simulink model "distributed_system"  (R2018a)
settings: Solver=VariableStepDiscrete  StartTime=0.0  StopTime=Inf  FixedStep=0.01  RelTol=1e-3  EnableMultiTasking=on
model workspace (MAT data in the model file):
  SL_ROS_VariableLengthArrays_MaxSizes.CommonInfo.ArrayTruncateAction = 'EmitWarning'
  SL_ROS_VariableLengthArrays_MaxSizes.MsgTypeMap = containers.Map
  SL_ROS_VariableLengthArrays_MaxSizes.MsgTypeMap.serialization.keys = {'sensor_msgs/Image', 'sensor_msgs/LaserScan'}
  SL_ROS_VariableLengthArrays_MaxSizes.MsgTypeMap.serialization.values{1}(1).PropertyName = 'Data'
  SL_ROS_VariableLengthArrays_MaxSizes.MsgTypeMap.serialization.values{1}(1).DataType = 'uint8'
  SL_ROS_VariableLengthArrays_MaxSizes.MsgTypeMap.serialization.values{1}(1).MaxLength = 691200
  SL_ROS_VariableLengthArrays_MaxSizes.MsgTypeMap.serialization.values{1}(2).PropertyName = 'Encoding'
  SL_ROS_VariableLengthArrays_MaxSizes.MsgTypeMap.serialization.values{1}(2).DataType = 'uint8'
  SL_ROS_VariableLengthArrays_MaxSizes.MsgTypeMap.serialization.values{1}(2).MaxLength = 128
  SL_ROS_VariableLengthArrays_MaxSizes.MsgTypeMap.serialization.values{2}(1).PropertyName = 'Intensities'
  SL_ROS_VariableLengthArrays_MaxSizes.MsgTypeMap.serialization.values{2}(1).DataType = 'single'
  SL_ROS_VariableLengthArrays_MaxSizes.MsgTypeMap.serialization.values{2}(1).MaxLength = 1081
  SL_ROS_VariableLengthArrays_MaxSizes.MsgTypeMap.serialization.values{2}(2).PropertyName = 'Ranges'
  SL_ROS_VariableLengthArrays_MaxSizes.MsgTypeMap.serialization.values{2}(2).DataType = 'single'
  SL_ROS_VariableLengthArrays_MaxSizes.MsgTypeMap.serialization.values{2}(2).MaxLength = 1081
  SL_ROS_VariableLengthArrays_MaxSizes.MsgTypeMap.serialization.uniformity = 0
  SL_ROS_VariableLengthArrays_MaxSizes.MsgTypeMap.serialization.keyType = 'char'
  SL_ROS_VariableLengthArrays_MaxSizes.MsgTypeMap.serialization.valueType = 'any'
undefined symbols (not defined in the file or in its folder): DiscIntNeverNeededParam, hz, Vector_
libraries: simulink x5, robotlib x4, sharedTrackingLibrary x4, aerolibanimutils x1
settings Model: Creator=The MathWorks, Inc.  LastModifiedBy=kevin
settings DataIOCC: LimitDataPoints=on  SaveFormat=Array
settings OptimizationCC: LifeSpan=Inf  MaxStackSize=64
settings DebuggingCC: SolverPrmCheckMsg=warning  SFUnexpectedBacktrackingDiag=warning  SFNoUnconditionalDefaultTransitionDiag=warning  SFExecutionAtInitializationDiag=none
settings HardwareCC: ProdBitPerLong=64  ProdHWDeviceType=Intel->x86-64 (Linux 64)  UseEmbeddedCoderFeatures=off
settings ModelReferenceCC: PropagateSignalLabelsOutOfModel=off
settings RTWCC: SystemTargetFile=ert.tlc  HardwareBoard=Robot Operating System (ROS)  TLCOptions=-aInlineSetEventsForThisBaseRateFcn=TLC_FALSE -aSuppressMultiTaskScheduler=TLC_FALSE -aRateBasedStepFcn=0  TemplateMakefile=ert_default_tmf  Toolchain=Catkin  TargetLang=C++
settings CodeAppCC: StateflowObjectComments=on
settings ERTTargetCC: MultiwordLength=2048  ERTCustomFileBanners=off  SupportContinuousTime=on  SupportNonInlinedSFcns=on  RemoveResetFunc=off  SupportVariableSizeSignals=on  ModelStepFunctionPrototypeControlCompliant=off  ConvertIfToSwitch=off  SuppressUnreachableDefaultCases=off
settings ConfigComp: CovMetricSettings=dw  CovHtmlReporting=on  CovSaveCumulativeToWorkspaceVar=on  CovSaveSingleToWorkspaceVar=on  CovExternalEMLEnable=off  CovSFcnEnable=off

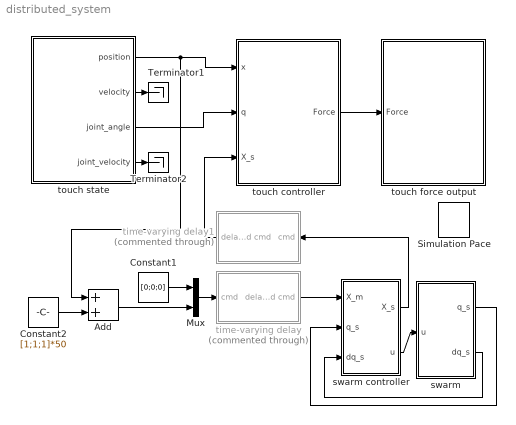
== system distributed_system ==
  Add : Sum
  Constant1 : Constant  Value=[0;0;0]
  Constant2 : Constant  Value=[1;1;1]*50
  Mux : Mux  Inputs=2
  Simulation Pace : aerolibanimutils/Simulation Pace  SimulationPace=1  SleepMode=MATLAB Thread  OutputPaceError=off  SampleTime=-1
  Terminator1 : Terminator
  Terminator2 : Terminator
  swarm : Subsystem
  swarm controller : Subsystem
  time-varying delay : Subsystem  Commented=through
  time-varying delay1 : Subsystem  Commented=through
  touch controller : Subsystem
  touch force output : Subsystem
  touch state : Subsystem
  wires:
  swarm/1(q_s) -> swarm controller/2(q_s)
  swarm/2(dq_s) -> swarm controller/3(dq_s)
  swarm controller/2(u) -> swarm/1(u)
  touch controller/1(Force) -> touch force output/1(Force)
  touch state/3(joint_angle) -> touch controller/2(q)
  swarm controller/1(X_s) -> time-varying delay1/1(cmd)
  Mux/1 -> time-varying delay/1(cmd)
  time-varying delay/1(delayed cmd) -> swarm controller/1(X_m)
  time-varying delay1/1(delayed cmd) -> touch controller/3(X_s)
  touch state/2(velocity) -> Terminator1/1
  touch state/4(joint_velocity) -> Terminator2/1
  Constant1/1 -> Mux/1
  Constant2/1 -> Add/2
  touch state/1(position) -> Add/1, touch controller/1(x)
  Add/1 -> Mux/2

== system distributed_system/swarm ==
  u : Inport
  Discrete-Time Integrator : DiscreteIntegrator  InitialCondition=zeros(18,1)  SampleTime=-1  ICPrevOutput=DiscIntNeverNeededParam  ICPrevScaledInput=DiscIntNeverNeededParam
  Discrete-Time Integrator1 : DiscreteIntegrator  InitialCondition=[1 0 0 0.7 0.7 0 -0.7 0.7 0 -1 0 0 -0.7 -0.7 0 0.7 -0.7 0].'  SampleTime=-1  ICPrevOutput=DiscIntNeverNeededParam  ICPrevScaledInput=DiscIntNeverNeededParam
  Subsystem1 : Subsystem
  q_s : Outport
  dq_s : Outport  Port=2
  wires:
  u/1 -> Discrete-Time Integrator/1
  Discrete-Time Integrator/1 -> Discrete-Time Integrator1/1, dq_s/1
  Discrete-Time Integrator1/1 -> q_s/1, Subsystem1/1(In1)

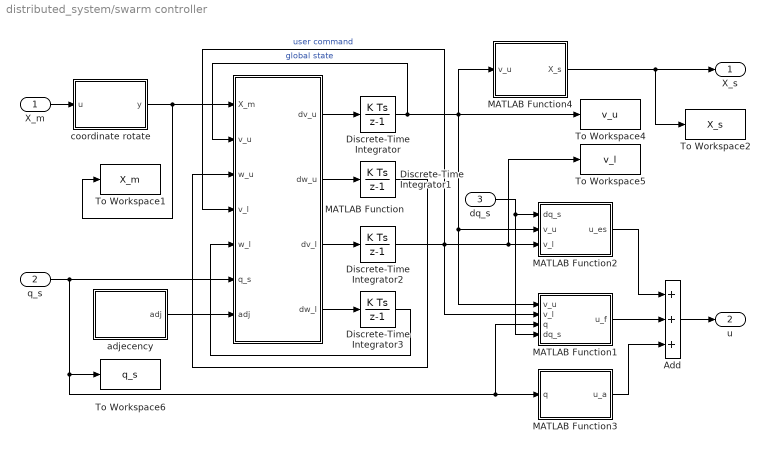
== system distributed_system/swarm controller ==
  X_m : Inport
  q_s : Inport  Port=2
  dq_s : Inport  Port=3
  Add : Sum  Inputs=+++
  Discrete-Time Integrator{,1..3} (4 alike) : DiscreteIntegrator  SampleTime=-1  ICPrevOutput=DiscIntNeverNeededParam  ICPrevScaledInput=DiscIntNeverNeededParam
  MATLAB Function : MATLAB Function  TreatAsAtomicUnit=on
  MATLAB Function1 : MATLAB Function  TreatAsAtomicUnit=on
  MATLAB Function2 : MATLAB Function  TreatAsAtomicUnit=on
  MATLAB Function3 : MATLAB Function  TreatAsAtomicUnit=on
  MATLAB Function4 : MATLAB Function  TreatAsAtomicUnit=on
  To Workspace1 : ToWorkspace  VariableName=X_m  SampleTime=-1
  To Workspace2 : ToWorkspace  VariableName=X_s  SampleTime=-1
  To Workspace4 : ToWorkspace  VariableName=v_u  SampleTime=-1
  To Workspace5 : ToWorkspace  VariableName=v_l  SampleTime=-1
  To Workspace6 : ToWorkspace  VariableName=q_s  SampleTime=-1
  adjecency : MATLAB Function  TreatAsAtomicUnit=on
  coordinate rotate : MATLAB Function  TreatAsAtomicUnit=on
  X_s : Outport
  u : Outport  Port=2
  wires:
  Discrete-Time Integrator1/1 -> MATLAB Function/3(w_u)
  q_s/1 -> MATLAB Function1/3(q), MATLAB Function3/1(q), To Workspace6/1, MATLAB Function/6(q_s)
  Discrete-Time Integrator3/1 -> MATLAB Function/5(w_l)
  Discrete-Time Integrator2/1 -> To Workspace5/1, MATLAB Function2/3(v_l), MATLAB Function1/2(v_l), MATLAB Function/4(v_l)  "user command"
  MATLAB Function/3(dv_l) -> Discrete-Time Integrator2/1
  MATLAB Function/4(dw_l) -> Discrete-Time Integrator3/1
  Add/1 -> u/1
  MATLAB Function/2(dw_u) -> Discrete-Time Integrator1/1
  Discrete-Time Integrator/1 -> To Workspace4/1, MATLAB Function4/1(v_u), MATLAB Function1/1(v_u), MATLAB Function2/2(v_u), MATLAB Function/2(v_u)  "global state"
  MATLAB Function/1(dv_u) -> Discrete-Time Integrator/1
  MATLAB Function3/1(u_a) -> Add/3
  dq_s/1 -> MATLAB Function1/4(dq_s), MATLAB Function2/1(dq_s)
  X_m/1 -> coordinate rotate/1(u)
  adjecency/1(adj) -> MATLAB Function/7(adj)
  MATLAB Function4/1(X_s) -> To Workspace2/1, X_s/1
  coordinate rotate/1(y) -> To Workspace1/1, MATLAB Function/1(X_m)
  MATLAB Function2/1(u_es) -> Add/1
  MATLAB Function1/1(u_f) -> Add/2

== system distributed_system/time-varying delay ==
  cmd : Inport
  Sine Wave : Sin  Amplitude=0.5  Bias=0.5  SampleTime=1/hz
  T_l : Scope
  Variable Time Delay : VariableTransportDelay  MaximumDelay=5
  delayed cmd : Outport
  wires:
  Sine Wave/1 -> Variable Time Delay/2, T_l/1
  Variable Time Delay/1 -> delayed cmd/1
  cmd/1 -> Variable Time Delay/1

== system distributed_system/time-varying delay1 ==
  cmd : Inport
  Sine Wave : Sin  Amplitude=0.5  Bias=0.5  SampleTime=1/hz
  T_l : Scope
  Variable Time Delay : VariableTransportDelay  MaximumDelay=5
  delayed cmd : Outport
  wires:
  cmd/1 -> Variable Time Delay/1
  Variable Time Delay/1 -> delayed cmd/1
  Sine Wave/1 -> T_l/1, Variable Time Delay/2

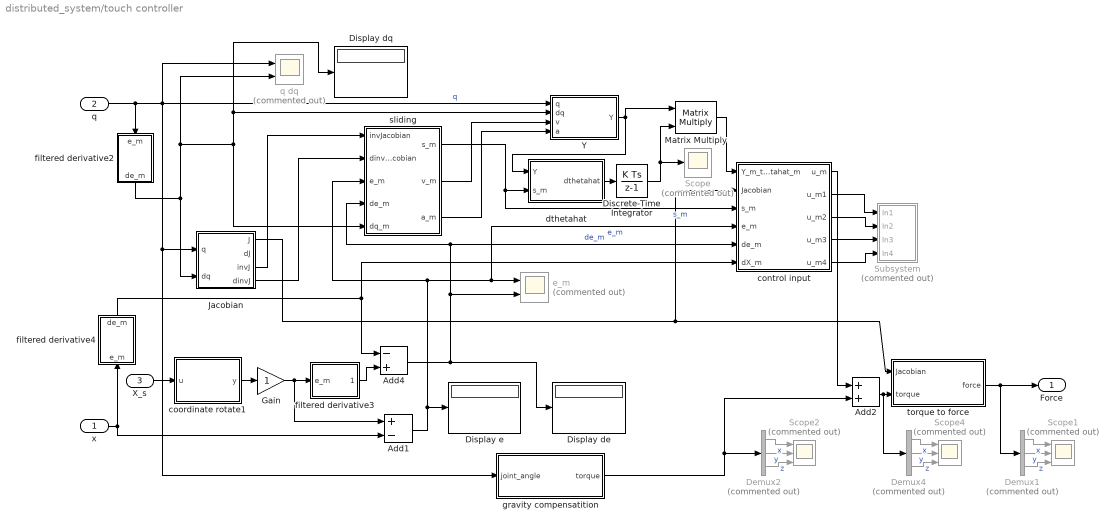
== system distributed_system/touch controller ==
  x : Inport
  q : Inport  Port=2
  X_s : Inport  Port=3
  Add1 : Sum  Inputs=+-
  Add2 : Sum
  Add4 : Sum  Inputs=-+
  Demux1 : Demux  Commented=on  Outputs=3
  Demux2 : Demux  Commented=on  Outputs=3
  Demux4 : Demux  Commented=on  Outputs=3
  Discrete-Time Integrator : DiscreteIntegrator  SampleTime=-1  ICPrevOutput=DiscIntNeverNeededParam  ICPrevScaledInput=DiscIntNeverNeededParam
  Display de : Display
  Display dq : Display
  Display e : Display
  Gain : Gain
  Jacobian : MATLAB Function  TreatAsAtomicUnit=on
  Matrix Multiply : Product  Multiplication=Matrix(*)
  Scope : Scope  Commented=on
  Scope1 : Scope  Commented=on  NumInputPorts=3
  Scope2 : Scope  Commented=on  NumInputPorts=3
  Scope4 : Scope  Commented=on  NumInputPorts=3
  Subsystem : Subsystem  Commented=on
  Y : MATLAB Function  TreatAsAtomicUnit=on
  control input : MATLAB Function  TreatAsAtomicUnit=on
  coordinate rotate1 : MATLAB Function  TreatAsAtomicUnit=on
  dthetahat : MATLAB Function  TreatAsAtomicUnit=on
  e_m : Scope  Commented=on  NumInputPorts=2
  filtered derivative2 : Subsystem
  filtered derivative3 : Subsystem
  filtered derivative4 : Subsystem
  gravity compensatition : MATLAB Function  TreatAsAtomicUnit=on
  q dq : Scope  Commented=on  NumInputPorts=2
  sliding : MATLAB Function  TreatAsAtomicUnit=on
  torque to force : MATLAB Function  TreatAsAtomicUnit=on
  Force : Outport
  wires:
  Jacobian/1(J) -> torque to force/1(Jacobian), control input/2(Jacobian)
  gravity compensatition/1(torque) -> Add2/2, Demux2/1
  torque to force/1(force) -> Demux1/1, Force/1
  Demux1/1 -> Scope1/1  "x"
  Demux1/3 -> Scope1/3  "z"
  Demux1/2 -> Scope1/2  "y"
  Demux2/2 -> Scope2/2  "y"
  Demux2/3 -> Scope2/3  "z"
  Demux2/1 -> Scope2/1  "x"
  sliding/1(s_m) -> control input/3(s_m), dthetahat/2(s_m)  "s_m"
  q/1 -> Y/1(q), q dq/1, gravity compensatition/1(joint_angle), Jacobian/1(q), filtered derivative2/1(e_m)  "q"
  dthetahat/1(dthetahat) -> Discrete-Time Integrator/1
  Y/1(Y) -> Matrix Multiply/1, dthetahat/1(Y)
  Discrete-Time Integrator/1 -> Scope/1, Matrix Multiply/2
  filtered derivative2/1(de_m) -> Jacobian/2(dq), Display dq/1, Y/2(dq), sliding/5(dq_m), q dq/2
  X_s/1 -> coordinate rotate1/1(u)
  Gain/1 -> filtered derivative3/1(e_m), Add1/1
  coordinate rotate1/1(y) -> Gain/1
  Add1/1 -> Display e/1, control input/4(e_m), e_m/1, sliding/3(e_m)  "e_m"
  Add4/1 -> Display de/1, e_m/2, control input/5(de_m), sliding/4(de_m)  "de_m"
  control input/1(u_m) -> Add2/1
  x/1 -> Add1/2, filtered derivative4/1(e_m)
  filtered derivative3/1(de_m) -> Add4/2
  filtered derivative4/1(de_m) -> control input/6(dX_m), Add4/1
  sliding/2(v_m) -> Y/3(v)
  sliding/3(a_m) -> Y/4(a)
  Jacobian/3(invJ) -> sliding/1(invJacobian)
  Jacobian/4(dinvJ) -> sliding/2(dinvJacobian)
  Matrix Multiply/1 -> control input/1(Y_m_thetahat_m)
  control input/2(u_m1) -> Subsystem/1(In1)
  control input/3(u_m2) -> Subsystem/2(In2)
  control input/4(u_m3) -> Subsystem/3(In3)
  control input/5(u_m4) -> Subsystem/4(In4)
  Demux4/2 -> Scope4/2  "y"
  Demux4/3 -> Scope4/3  "z"
  Demux4/1 -> Scope4/1  "x"
  Add2/1 -> Demux4/1, torque to force/2(torque)

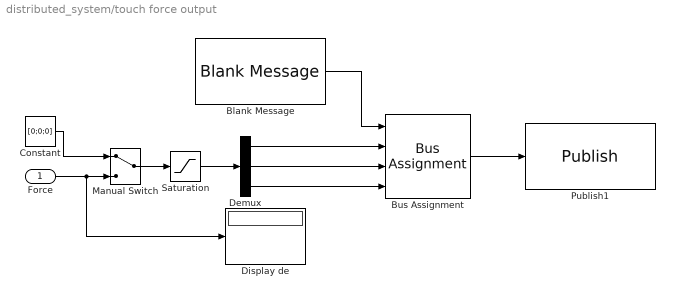
== system distributed_system/touch force output ==
  Force : Inport
  Blank Message : robotlib/Blank Message  SourceLibraryInfo=This block requires Robotics System Toolbox  messageType=geometry_msgs/Vector3Stamped  SampleTime=1/hz
      settings: SourceProductBaseCode=RO
  Bus Assignment : BusAssignment  DialogController=Simulink.DDGSource_BusAssignment  AssignedSignals=Vector_.X,Vector_.Y,Vector_.Z
  Constant : Constant  Value=[0;0;0]  SampleTime=1/hz
  Demux : Demux  Outputs=3
  Display de : Display
  Manual Switch : ManualSwitch
  Publish1 : robotlib/Publish  SourceLibraryInfo=This block requires Robotics System Toolbox  topicSource=Select from ROS network  topic=/touch_1/touch_force  messageType=geometry_msgs/Vector3Stamped  messageQueueLength=105
      settings: SourceProductBaseCode=RO
  Saturation : Saturate  UpperLimit=[1;1;1]*5  LowerLimit=[-1;-1;-1]*5
  wires:
  Demux/2 -> Bus Assignment/3
  Demux/1 -> Bus Assignment/2
  Demux/3 -> Bus Assignment/4
  Bus Assignment/1 -> Publish1/1
  Blank Message/1 -> Bus Assignment/1
  Force/1 -> Display de/1, Manual Switch/2
  Constant/1 -> Manual Switch/1
  Manual Switch/1 -> Saturation/1
  Saturation/1 -> Demux/1

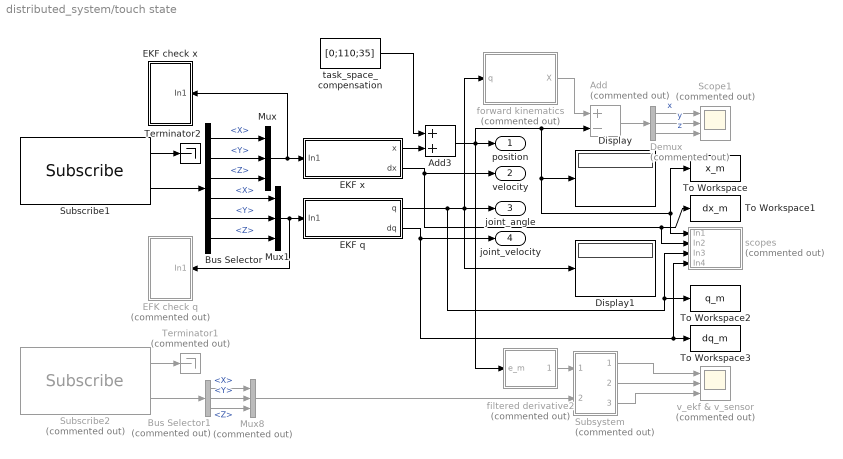
== system distributed_system/touch state ==
  Add : Sum  Commented=on  Inputs=+-
  Add3 : Sum
  Bus Selector : BusSelector  DialogController=Simulink.DDGSource_BusSelector  OutputSignals=Twist.Linear.X,Twist.Linear.Y,Twist.Linear.Z,Twist.Angular.X,Twist.Angular.Y,Twist.Angular.Z
  Bus Selector1 : BusSelector  Commented=on  DialogController=Simulink.DDGSource_BusSelector  OutputSignals=Vector_.X,Vector_.Y,Vector_.Z
  Demux : Demux  Commented=on  Outputs=3
  Display : Display
  Display1 : Display
  EFK check q : Subsystem  Commented=on
  EKF check x : Subsystem
  EKF q : Subsystem
  EKF x : Subsystem
  Mux : Mux  Inputs=3
  Mux1 : Mux  Inputs=3
  Mux8 : Mux  Commented=on  Inputs=3
  Scope1 : Scope  Commented=on  NumInputPorts=3
  Subscribe1 : robotlib/Subscribe  SourceLibraryInfo=This block requires Robotics System Toolbox  topicSource=Select from ROS network  topic=/touch_1/touch_state  messageType=geometry_msgs/TwistStamped  sampleTime=1/hz  messageQueueLength=51
      settings: SourceProductBaseCode=RO
  Subscribe2 : robotlib/Subscribe  Commented=on  SourceLibraryInfo=This block requires Robotics System Toolbox  topicSource=Select from ROS network  topic=/touch_1/touch_vel_hd  messageType=geometry_msgs/Vector3Stamped  sampleTime=1/hz  messageQueueLength=51
      settings: SourceProductBaseCode=RO
  Subsystem : Subsystem  Commented=on
  Terminator1 : Terminator  Commented=on
  Terminator2 : Terminator
  To Workspace : ToWorkspace  VariableName=x_m  SampleTime=-1
  To Workspace1 : ToWorkspace  VariableName=dx_m  SampleTime=-1
  To Workspace2 : ToWorkspace  VariableName=q_m  SampleTime=-1
  To Workspace3 : ToWorkspace  VariableName=dq_m  SampleTime=-1
  filtered derivative2 : Subsystem  Commented=on
  forward kinematics : MATLAB Function  Commented=on  TreatAsAtomicUnit=on
  scopes : Subsystem  Commented=on
  task_space_compensation : Constant  Value=[0;110;35]  SampleTime=1/hz
  v_ekf & v_sensor : Scope  Commented=on  NumInputPorts=3
  position : Outport
  velocity : Outport  Port=2
  joint_angle : Outport  Port=3
  joint_velocity : Outport  Port=4
  wires:
  Subscribe1/2 -> Bus Selector/1
  Bus Selector/1 -> Mux/1  "<X>"
  Bus Selector/5 -> Mux1/2  "<Y>"
  Bus Selector/4 -> Mux1/1  "<X>"
  Bus Selector/6 -> Mux1/3  "<Z>"
  Add/1 -> Demux/1
  Demux/3 -> Scope1/3  "z"
  Demux/1 -> Scope1/1  "x"
  Demux/2 -> Scope1/2  "y"
  Subscribe2/1 -> Terminator1/1
  Subscribe1/1 -> Terminator2/1
  Mux1/1 -> EKF q/1(In1), EFK check q/1(In1)
  Subscribe2/2 -> Bus Selector1/1
  forward kinematics/1(X) -> Add/1
  Bus Selector/2 -> Mux/2  "<Y>"
  Bus Selector/3 -> Mux/3  "<Z>"
  Mux/1 -> EKF x/1(In1), EKF check x/1(In1)
  EKF q/1(q) -> scopes/3(In3), To Workspace2/1, Display1/1, joint_angle/1, forward kinematics/1(q)
  EKF x/2(dx) -> To Workspace1/1, scopes/2(In2), velocity/1
  EKF q/2(dq) -> scopes/4(In4), To Workspace3/1, joint_velocity/1
  Subsystem/1(Out1) -> v_ekf & v_sensor/1
  Subsystem/2(Out2) -> v_ekf & v_sensor/2
  Subsystem/3(Out3) -> v_ekf & v_sensor/3
  Bus Selector1/1 -> Mux8/1  "<X>"
  Bus Selector1/2 -> Mux8/2  "<Y>"
  Bus Selector1/3 -> Mux8/3  "<Z>"
  Mux8/1 -> Subsystem/2(In2)
  filtered derivative2/1(de_m) -> Subsystem/1(In1)
  EKF x/1(x) -> Add3/2
  task_space_compensation/1 -> Add3/1
  Add3/1 -> filtered derivative2/1(e_m), scopes/1(In1), To Workspace/1, Display/1, Add/2, position/1

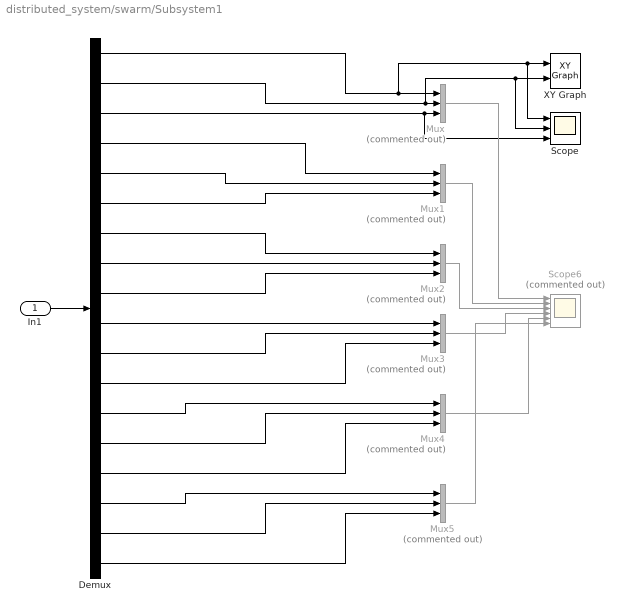
== system distributed_system/swarm/Subsystem1 ==
  In1 : Inport
  Demux : Demux  Outputs=18
  Mux{,1..5} (6 alike) : Mux  Commented=on  Inputs=3
  Scope : Scope  NumInputPorts=3
  Scope6 : Scope  Commented=on  NumInputPorts=6
  XY Graph : simulink/Sinks/XY Graph  xmin=-10  xmax=10  ymin=-10  ymax=10  st=-1
  wires:
  In1/1 -> Demux/1
  Demux/3 -> Scope/3, Mux/3
  Demux/2 -> Scope/2, XY Graph/2, Mux/2
  Demux/1 -> Scope/1, XY Graph/1, Mux/1
  Demux/5 -> Mux1/2
  Demux/6 -> Mux1/3
  Demux/4 -> Mux1/1
  Demux/8 -> Mux2/2
  Demux/7 -> Mux2/1
  Demux/9 -> Mux2/3
  Demux/10 -> Mux3/1
  Demux/11 -> Mux3/2
  Demux/12 -> Mux3/3
  Demux/13 -> Mux4/1
  Demux/14 -> Mux4/2
  Demux/15 -> Mux4/3
  Demux/16 -> Mux5/1
  Demux/17 -> Mux5/2
  Demux/18 -> Mux5/3
  Mux/1 -> Scope6/1
  Mux1/1 -> Scope6/2
  Mux2/1 -> Scope6/3
  Mux3/1 -> Scope6/4
  Mux4/1 -> Scope6/5
  Mux5/1 -> Scope6/6

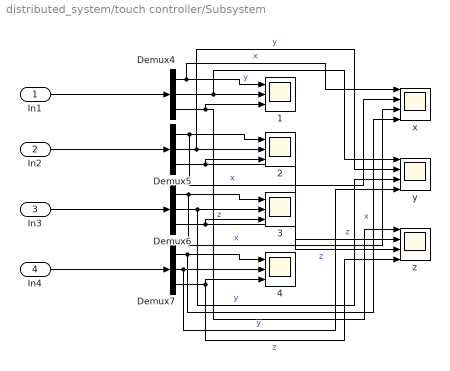
== system distributed_system/touch controller/Subsystem ==
  In1 : Inport
  In2 : Inport  Port=2
  In3 : Inport  Port=3
  In4 : Inport  Port=4
  {1..4} (4 alike) : Scope  NumInputPorts=3
  Demux{4..7} (4 alike) : Demux  Outputs=3
  x : Scope  NumInputPorts=4
  y : Scope  NumInputPorts=4
  z : Scope  NumInputPorts=4
  wires:
  Demux5/1 -> x/2, 2/1  "x"
  Demux6/3 -> 3/3, z/3  "z"
  Demux6/1 -> 3/1, x/3  "x"
  In4/1 -> Demux7/1
  Demux5/3 -> z/2, 2/3  "z"
  Demux4/3 -> z/1, 1/3  "z"
  Demux6/2 -> 3/2, y/3  "y"
  Demux5/2 -> y/2, 2/2  "y"
  Demux4/2 -> y/1, 1/2  "y"
  Demux4/1 -> x/1, 1/1  "x"
  Demux7/1 -> x/4, 4/1  "x"
  Demux7/3 -> z/4, 4/3  "z"
  In2/1 -> Demux5/1
  Demux7/2 -> y/4, 4/2  "y"
  In3/1 -> Demux6/1
  In1/1 -> Demux4/1

== system distributed_system/touch controller/filtered derivative2 ==
  e_m : Inport
  Filter : DiscreteIntegrator  DisableCoverage=on  SampleTime=-1  ICPrevOutput=DiscIntNeverNeededParam  ICPrevScaledInput=DiscIntNeverNeededParam
  Filter Coefficient : Gain  Gain=100
  SumD : Sum  DisableCoverage=on  Inputs=|+-
  de_m : Outport
  wires:
  Filter Coefficient/1 -> de_m/1, Filter/1
  Filter/1 -> SumD/2
  SumD/1 -> Filter Coefficient/1
  e_m/1 -> SumD/1

== system distributed_system/touch controller/filtered derivative3 ==
  e_m : Inport
  Filter : DiscreteIntegrator  DisableCoverage=on  SampleTime=-1  ICPrevOutput=DiscIntNeverNeededParam  ICPrevScaledInput=DiscIntNeverNeededParam
  Filter Coefficient : Gain  Gain=100
  SumD : Sum  DisableCoverage=on  Inputs=|+-
  de_m : Outport
  wires:
  Filter Coefficient/1 -> de_m/1, Filter/1
  Filter/1 -> SumD/2
  SumD/1 -> Filter Coefficient/1
  e_m/1 -> SumD/1

== system distributed_system/touch controller/filtered derivative4 ==
  e_m : Inport
  Filter : DiscreteIntegrator  DisableCoverage=on  SampleTime=-1  ICPrevOutput=DiscIntNeverNeededParam  ICPrevScaledInput=DiscIntNeverNeededParam
  Filter Coefficient : Gain  Gain=100
  SumD : Sum  DisableCoverage=on  Inputs=|+-
  de_m : Outport
  wires:
  e_m/1 -> SumD/1
  SumD/1 -> Filter Coefficient/1
  Filter/1 -> SumD/2
  Filter Coefficient/1 -> Filter/1, de_m/1

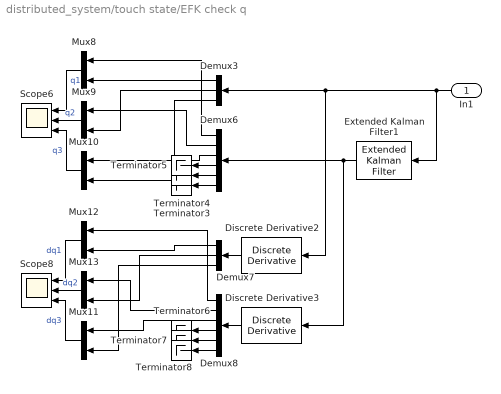
== system distributed_system/touch state/EFK check q ==
  In1 : Inport
  Demux3 : Demux  Outputs=3
  Demux6 : Demux  Outputs=6
  Demux7 : Demux  Outputs=3
  Demux8 : Demux  Outputs=6
  Discrete Derivative2 : simulink/Discrete/Discrete Derivative  gainval=1.0  ICPrevScaledInput=0.0  OutMin=[]  OutMax=[]  OutDataType=fixdt(1, 16)  OutScaling=2^-10  DoSatur=off
  Discrete Derivative3 : simulink/Discrete/Discrete Derivative  gainval=1.0  ICPrevScaledInput=0.0  OutMin=[]  OutMax=[]  OutDataType=fixdt(1, 16)  OutScaling=2^-10  DoSatur=off
  Extended Kalman Filter1 : sharedTrackingLibrary/Extended Kalman Filter  StateTransitionFcn=myStateTransitionFcn  HasStateTransitionJacobianFcn=off  HasAdditiveProcessNoise=Additive  ProcessNoise=diag([0 0 0 1 1 1]*5e-2)  HasTimeVaryingProcessNoise=off  HasStateTransitionFcnExtraArgument=0  InitialState=[0 0 0 0 0 0]  InitialStateCovariance=diag([1 1 1 1 1 1]*1e-1)  MeasurementFcn1=myMeasurementFcn  HasMeasurementJacobianFcn1=off  HasMeasurementEnablePort1=off  HasAdditiveMeasurementNoise1=Additive  MeasurementNoise1=diag([1;1;1]*3e-3)  HasTimeVaryingMeasurementNoise1=off  HasMeasurementFcnExtraArgument1=0  MeasurementFcn2=myMeasurementFcn  HasMeasurementJacobianFcn2=off  HasMeasurementEnablePort2=off  HasAdditiveMeasurementNoise2=Additive  MeasurementNoise2=1  HasTimeVaryingMeasurementNoise2=off  HasMeasurementFcnExtraArgument2=0  MeasurementFcn3=myMeasurementFcn  HasMeasurementJacobianFcn3=off  HasMeasurementEnablePort3=off  HasAdditiveMeasurementNoise3=Additive  MeasurementNoise3=1  HasTimeVaryingMeasurementNoise3=off  HasMeasurementFcnExtraArgument3=0  MeasurementFcn4=myMeasurementFcn  HasMeasurementJacobianFcn4=off  HasMeasurementEnablePort4=off  HasAdditiveMeasurementNoise4=Additive  MeasurementNoise4=1  HasTimeVaryingMeasurementNoise4=off  HasMeasurementFcnExtraArgument4=0  MeasurementFcn5=myMeasurementFcn  HasMeasurementJacobianFcn5=off  HasMeasurementEnablePort5=off  HasAdditiveMeasurementNoise5=Additive  MeasurementNoise5=1  HasTimeVaryingMeasurementNoise5=off  HasMeasurementFcnExtraArgument5=0  EnableMultirate=off  StateTransitionFcnSampleTime=1  MeasurementFcn1SampleTime=1  MeasurementFcn2SampleTime=1  MeasurementFcn3SampleTime=1  MeasurementFcn4SampleTime=1  MeasurementFcn5SampleTime=1  UseCurrentEstimator=on  OutputStateCovariance=off  DataType=double  SampleTime=1/hz  NumberOfMeasurements=1
      settings: SourceProductName=Control System Toolbox  SourceProductBaseCode=CT
  Mux{8..13} (6 alike) : Mux  Inputs=2
  Scope6 : Scope  NumInputPorts=3
  Scope8 : Scope  NumInputPorts=3
  Terminator{3..8} (6 alike) : Terminator
  wires:
  In1/1 -> Discrete Derivative2/1, Demux3/1, Extended Kalman Filter1/1
  Demux3/1 -> Mux8/2
  Demux8/3 -> Mux11/1
  Demux3/2 -> Mux9/2
  Mux11/1 -> Scope8/3  "dq3"
  Mux12/1 -> Scope8/1  "dq1"
  Demux3/3 -> Mux10/2
  Demux7/2 -> Mux13/2
  Demux6/4 -> Terminator5/1
  Demux6/2 -> Mux9/1
  Demux8/5 -> Terminator7/1
  Demux8/4 -> Terminator6/1
  Mux13/1 -> Scope8/2  "dq2"
  Demux8/1 -> Mux12/1
  Mux9/1 -> Scope6/2  "q2"
  Mux10/1 -> Scope6/3  "q3"
  Demux6/3 -> Mux10/1
  Mux8/1 -> Scope6/1  "q1"
  Demux8/2 -> Mux13/1
  Demux6/1 -> Mux8/1
  Demux8/6 -> Terminator8/1
  Extended Kalman Filter1/1 -> Demux6/1, Discrete Derivative3/1
  Demux6/5 -> Terminator4/1
  Demux7/1 -> Mux12/2
  Demux7/3 -> Mux11/2
  Discrete Derivative2/1 -> Demux7/1
  Demux6/6 -> Terminator3/1
  Discrete Derivative3/1 -> Demux8/1

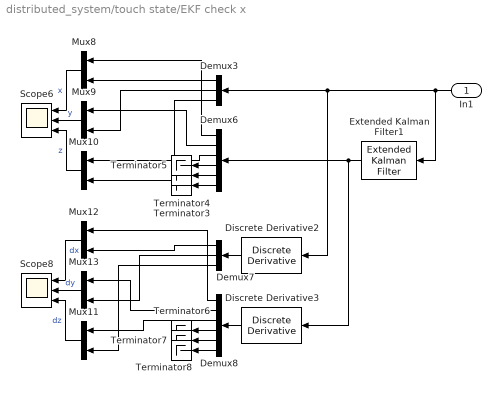
== system distributed_system/touch state/EKF check x ==
  In1 : Inport
  Demux3 : Demux  Outputs=3
  Demux6 : Demux  Outputs=6
  Demux7 : Demux  Outputs=3
  Demux8 : Demux  Outputs=6
  Discrete Derivative2 : simulink/Discrete/Discrete Derivative  gainval=1.0  ICPrevScaledInput=0.0  OutMin=[]  OutMax=[]  OutDataType=fixdt(1, 16)  OutScaling=2^-10  DoSatur=off
  Discrete Derivative3 : simulink/Discrete/Discrete Derivative  gainval=1.0  ICPrevScaledInput=0.0  OutMin=[]  OutMax=[]  OutDataType=fixdt(1, 16)  OutScaling=2^-10  DoSatur=off
  Extended Kalman Filter1 : sharedTrackingLibrary/Extended Kalman Filter  StateTransitionFcn=myStateTransitionFcn  HasStateTransitionJacobianFcn=off  HasAdditiveProcessNoise=Additive  ProcessNoise=diag([0 0 0 1 1 1]*5e-2)  HasTimeVaryingProcessNoise=off  HasStateTransitionFcnExtraArgument=0  InitialState=[0 0 0 0 0 0]  InitialStateCovariance=diag([1 1 1 1 1 1]*1e-1)  MeasurementFcn1=myMeasurementFcn  HasMeasurementJacobianFcn1=off  HasMeasurementEnablePort1=off  HasAdditiveMeasurementNoise1=Additive  MeasurementNoise1=diag([1;1;1]*3e-3)  HasTimeVaryingMeasurementNoise1=off  HasMeasurementFcnExtraArgument1=0  MeasurementFcn2=myMeasurementFcn  HasMeasurementJacobianFcn2=off  HasMeasurementEnablePort2=off  HasAdditiveMeasurementNoise2=Additive  MeasurementNoise2=1  HasTimeVaryingMeasurementNoise2=off  HasMeasurementFcnExtraArgument2=0  MeasurementFcn3=myMeasurementFcn  HasMeasurementJacobianFcn3=off  HasMeasurementEnablePort3=off  HasAdditiveMeasurementNoise3=Additive  MeasurementNoise3=1  HasTimeVaryingMeasurementNoise3=off  HasMeasurementFcnExtraArgument3=0  MeasurementFcn4=myMeasurementFcn  HasMeasurementJacobianFcn4=off  HasMeasurementEnablePort4=off  HasAdditiveMeasurementNoise4=Additive  MeasurementNoise4=1  HasTimeVaryingMeasurementNoise4=off  HasMeasurementFcnExtraArgument4=0  MeasurementFcn5=myMeasurementFcn  HasMeasurementJacobianFcn5=off  HasMeasurementEnablePort5=off  HasAdditiveMeasurementNoise5=Additive  MeasurementNoise5=1  HasTimeVaryingMeasurementNoise5=off  HasMeasurementFcnExtraArgument5=0  EnableMultirate=off  StateTransitionFcnSampleTime=1  MeasurementFcn1SampleTime=1  MeasurementFcn2SampleTime=1  MeasurementFcn3SampleTime=1  MeasurementFcn4SampleTime=1  MeasurementFcn5SampleTime=1  UseCurrentEstimator=on  OutputStateCovariance=off  DataType=double  SampleTime=1/hz  NumberOfMeasurements=1
      settings: SourceProductName=Control System Toolbox  SourceProductBaseCode=CT
  Mux{8..13} (6 alike) : Mux  Inputs=2
  Scope6 : Scope  NumInputPorts=3
  Scope8 : Scope  NumInputPorts=3
  Terminator{3..8} (6 alike) : Terminator
  wires:
  Discrete Derivative3/1 -> Demux8/1
  Demux6/6 -> Terminator3/1
  Discrete Derivative2/1 -> Demux7/1
  Demux7/3 -> Mux11/2
  Demux7/1 -> Mux12/2
  Demux6/5 -> Terminator4/1
  Extended Kalman Filter1/1 -> Demux6/1, Discrete Derivative3/1
  Demux8/6 -> Terminator8/1
  Demux6/1 -> Mux8/1
  Demux8/2 -> Mux13/1
  Mux8/1 -> Scope6/1  "x"
  Demux6/3 -> Mux10/1
  Mux10/1 -> Scope6/3  "z"
  Mux9/1 -> Scope6/2  "y"
  Demux8/1 -> Mux12/1
  Mux13/1 -> Scope8/2  "dy"
  Demux8/4 -> Terminator6/1
  Demux8/5 -> Terminator7/1
  Demux6/2 -> Mux9/1
  Demux6/4 -> Terminator5/1
  Demux7/2 -> Mux13/2
  Demux3/3 -> Mux10/2
  Mux12/1 -> Scope8/1  "dx"
  Mux11/1 -> Scope8/3  "dz"
  Demux3/2 -> Mux9/2
  Demux8/3 -> Mux11/1
  Demux3/1 -> Mux8/2
  In1/1 -> Extended Kalman Filter1/1, Demux3/1, Discrete Derivative2/1

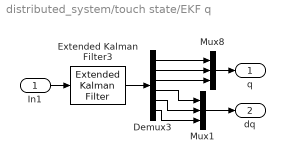
== system distributed_system/touch state/EKF q ==
  In1 : Inport
  Demux3 : Demux  Outputs=6
  Extended Kalman Filter3 : sharedTrackingLibrary/Extended Kalman Filter  StateTransitionFcn=myStateTransitionFcn  HasStateTransitionJacobianFcn=off  HasAdditiveProcessNoise=Additive  ProcessNoise=diag([0 0 0 1 1 1]*5e-2)  HasTimeVaryingProcessNoise=off  HasStateTransitionFcnExtraArgument=0  InitialState=[0 0 0 0 0 0]  InitialStateCovariance=diag([1 1 1 1 1 1]*1e-1)  MeasurementFcn1=myMeasurementFcn  HasMeasurementJacobianFcn1=off  HasMeasurementEnablePort1=off  HasAdditiveMeasurementNoise1=Additive  MeasurementNoise1=diag([1;1;1]*3e-3)  HasTimeVaryingMeasurementNoise1=off  HasMeasurementFcnExtraArgument1=0  MeasurementFcn2=myMeasurementFcn  HasMeasurementJacobianFcn2=off  HasMeasurementEnablePort2=off  HasAdditiveMeasurementNoise2=Additive  MeasurementNoise2=1  HasTimeVaryingMeasurementNoise2=off  HasMeasurementFcnExtraArgument2=0  MeasurementFcn3=myMeasurementFcn  HasMeasurementJacobianFcn3=off  HasMeasurementEnablePort3=off  HasAdditiveMeasurementNoise3=Additive  MeasurementNoise3=1  HasTimeVaryingMeasurementNoise3=off  HasMeasurementFcnExtraArgument3=0  MeasurementFcn4=myMeasurementFcn  HasMeasurementJacobianFcn4=off  HasMeasurementEnablePort4=off  HasAdditiveMeasurementNoise4=Additive  MeasurementNoise4=1  HasTimeVaryingMeasurementNoise4=off  HasMeasurementFcnExtraArgument4=0  MeasurementFcn5=myMeasurementFcn  HasMeasurementJacobianFcn5=off  HasMeasurementEnablePort5=off  HasAdditiveMeasurementNoise5=Additive  MeasurementNoise5=1  HasTimeVaryingMeasurementNoise5=off  HasMeasurementFcnExtraArgument5=0  EnableMultirate=off  StateTransitionFcnSampleTime=1  MeasurementFcn1SampleTime=1  MeasurementFcn2SampleTime=1  MeasurementFcn3SampleTime=1  MeasurementFcn4SampleTime=1  MeasurementFcn5SampleTime=1  UseCurrentEstimator=on  OutputStateCovariance=off  DataType=double  SampleTime=1/hz  NumberOfMeasurements=1
      settings: SourceProductName=Control System Toolbox  SourceProductBaseCode=CT
  Mux1 : Mux  Inputs=3
  Mux8 : Mux  Inputs=3
  q : Outport
  dq : Outport  Port=2
  wires:
  Mux8/1 -> q/1
  Demux3/6 -> Mux1/3
  Demux3/2 -> Mux8/2
  Demux3/3 -> Mux8/3
  Demux3/1 -> Mux8/1
  In1/1 -> Extended Kalman Filter3/1
  Demux3/4 -> Mux1/1
  Extended Kalman Filter3/1 -> Demux3/1
  Demux3/5 -> Mux1/2
  Mux1/1 -> dq/1

== system distributed_system/touch state/EKF x ==
  In1 : Inport
  Demux3 : Demux  Outputs=6
  Extended Kalman Filter3 : sharedTrackingLibrary/Extended Kalman Filter  StateTransitionFcn=myStateTransitionFcn  HasStateTransitionJacobianFcn=off  HasAdditiveProcessNoise=Additive  ProcessNoise=diag([0 0 0 1 1 1]*5e-2)  HasTimeVaryingProcessNoise=off  HasStateTransitionFcnExtraArgument=0  InitialState=[4 -110 -35 0 0 0]  InitialStateCovariance=diag([2 1 2 1 1 1])  MeasurementFcn1=myMeasurementFcn  HasMeasurementJacobianFcn1=off  HasMeasurementEnablePort1=off  HasAdditiveMeasurementNoise1=Additive  MeasurementNoise1=diag([1;1;1]*3e-3)  HasTimeVaryingMeasurementNoise1=off  HasMeasurementFcnExtraArgument1=0  MeasurementFcn2=myMeasurementFcn  HasMeasurementJacobianFcn2=off  HasMeasurementEnablePort2=off  HasAdditiveMeasurementNoise2=Additive  MeasurementNoise2=1  HasTimeVaryingMeasurementNoise2=off  HasMeasurementFcnExtraArgument2=0  MeasurementFcn3=myMeasurementFcn  HasMeasurementJacobianFcn3=off  HasMeasurementEnablePort3=off  HasAdditiveMeasurementNoise3=Additive  MeasurementNoise3=1  HasTimeVaryingMeasurementNoise3=off  HasMeasurementFcnExtraArgument3=0  MeasurementFcn4=myMeasurementFcn  HasMeasurementJacobianFcn4=off  HasMeasurementEnablePort4=off  HasAdditiveMeasurementNoise4=Additive  MeasurementNoise4=1  HasTimeVaryingMeasurementNoise4=off  HasMeasurementFcnExtraArgument4=0  MeasurementFcn5=myMeasurementFcn  HasMeasurementJacobianFcn5=off  HasMeasurementEnablePort5=off  HasAdditiveMeasurementNoise5=Additive  MeasurementNoise5=1  HasTimeVaryingMeasurementNoise5=off  HasMeasurementFcnExtraArgument5=0  EnableMultirate=off  StateTransitionFcnSampleTime=1  MeasurementFcn1SampleTime=1  MeasurementFcn2SampleTime=1  MeasurementFcn3SampleTime=1  MeasurementFcn4SampleTime=1  MeasurementFcn5SampleTime=1  UseCurrentEstimator=on  OutputStateCovariance=off  DataType=double  SampleTime=1/hz  NumberOfMeasurements=1
      settings: SourceProductName=Control System Toolbox  SourceProductBaseCode=CT
  Mux1 : Mux  Inputs=3
  Mux8 : Mux  Inputs=3
  x : Outport
  dx : Outport  Port=2
  wires:
  Demux3/5 -> Mux1/2
  Extended Kalman Filter3/1 -> Demux3/1
  Demux3/4 -> Mux1/1
  In1/1 -> Extended Kalman Filter3/1
  Demux3/1 -> Mux8/1
  Demux3/3 -> Mux8/3
  Demux3/2 -> Mux8/2
  Demux3/6 -> Mux1/3
  Mux8/1 -> x/1
  Mux1/1 -> dx/1

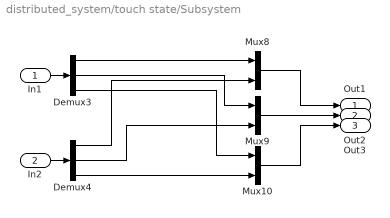
== system distributed_system/touch state/Subsystem ==
  In1 : Inport
  In2 : Inport  Port=2
  Demux3 : Demux  Outputs=3
  Demux4 : Demux  Outputs=3
  Mux10 : Mux  Inputs=2
  Mux8 : Mux  Inputs=2
  Mux9 : Mux  Inputs=2
  Out1 : Outport
  Out2 : Outport  Port=2
  Out3 : Outport  Port=3
  wires:
  In2/1 -> Demux4/1
  Demux4/2 -> Mux9/2
  Demux3/1 -> Mux8/1
  Demux4/1 -> Mux8/2
  Demux3/3 -> Mux10/1
  Demux3/2 -> Mux9/1
  Mux10/1 -> Out3/1
  Demux4/3 -> Mux10/2
  Mux8/1 -> Out1/1
  Mux9/1 -> Out2/1
  In1/1 -> Demux3/1

== system distributed_system/touch state/filtered derivative2 ==
  e_m : Inport
  Filter : DiscreteIntegrator  DisableCoverage=on  SampleTime=-1  ICPrevOutput=DiscIntNeverNeededParam  ICPrevScaledInput=DiscIntNeverNeededParam
  Filter Coefficient : Gain  Gain=100
  SumD : Sum  DisableCoverage=on  Inputs=|+-
  de_m : Outport
  wires:
  Filter Coefficient/1 -> de_m/1, Filter/1
  Filter/1 -> SumD/2
  SumD/1 -> Filter Coefficient/1
  e_m/1 -> SumD/1

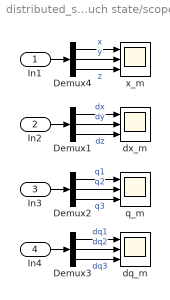
== system distributed_system/touch state/scopes ==
  In1 : Inport
  In2 : Inport  Port=2
  In3 : Inport  Port=3
  In4 : Inport  Port=4
  Demux{1..4} (4 alike) : Demux  Outputs=3
  dq_m : Scope  NumInputPorts=3
  dx_m : Scope  NumInputPorts=3
  q_m : Scope  NumInputPorts=3
  x_m : Scope  NumInputPorts=3
  wires:
  Demux3/1 -> dq_m/1  "dq1"
  Demux3/3 -> dq_m/3  "dq3"
  Demux4/1 -> x_m/1  "x"
  In3/1 -> Demux2/1
  Demux4/3 -> x_m/3  "z"
  Demux4/2 -> x_m/2  "y"
  In1/1 -> Demux4/1
  In2/1 -> Demux1/1
  In4/1 -> Demux3/1
  Demux1/3 -> dx_m/3  "dz"
  Demux1/1 -> dx_m/1  "dx"
  Demux3/2 -> dq_m/2  "dq2"
  Demux2/3 -> q_m/3  "q3"
  Demux1/2 -> dx_m/2  "dy"
  Demux2/1 -> q_m/1  "q1"
  Demux2/2 -> q_m/2  "q2"

== matlab function distributed_system/touch controller/torque to force ==
  data: Jacobian input; torque input; force output
function force = fcn(Jacobian, torque)

force = pinv(Jacobian).'*torque;

== matlab function distributed_system/touch controller/gravity compensatition ==
  data: joint_angle input; torque output
function torque = fcn(joint_angle)
q1 = joint_angle(1);
q2 = joint_angle(2);
q3 = joint_angle(3);
c1 = 85;
c2 = 70;

result = [0;c1*sin(q2+q3)+c2*cos(q2);c1*sin(q2+q3)];
% if result(2) < 0
%     result(2) = 0;
% end
torque = result;

== matlab function distributed_system/touch state/forward kinematics ==
  data: q input; X output
function X = fcn(q)
%#codegen

l1=133;
l2=133;

q1 = q(1);
q2 = q(2);
q3 = q(3);

s1 = sin(q1);
s2 = sin(q2);
s3 = sin(q3);

c1 = cos(q1);
c2 = cos(q2);
c3 = cos(q3);

X1 = -l1*s1*c2 - l2*s1*s2*c3 - l2*s1*c2*s3;
X2 = l1*s2 - l2*c2*c3 + l2*s2*s3 + l2;
X3 = l1*c1*c2 - l1 + l2*c1*s2*c3 + l2*c1*c2*s3;

X = [ X1;
      X2;
      X3];

== matlab function distributed_system/swarm controller/MATLAB Function ==
  data: X_m input; v_u input; dv_u output; dw_u output; w_u input; v_l input; w_l input; q_s input; adj input; dv_l output; dw_l output
function [dv_u,dw_u, dv_l, dw_l] = Estimator(X_m, v_u, w_u, v_l, w_l, q_s, adj)
SlaveRobotNum = 6;
SlaveRobotDOF = 3;
gamma = 1;
rho = diag([1;1;1;0.02;0.02;0.02]);
leader = 1;
k_i = 10;

dv_u = zeros(length(q_s),1);
dw_u = zeros(length(q_s),1);
dv_l = zeros(length(X_m)*SlaveRobotNum,1);
dw_l = zeros(length(X_m)*SlaveRobotNum,1);
delta = zeros(SlaveRobotNum,1);
delta(leader) = 1;

for i = 1 : SlaveRobotNum   %robot number
    %index
    i1 = (i-1) * SlaveRobotDOF + 1;
    i1e = i1 + SlaveRobotDOF - 1;
    i3 = (i-1) * length(X_m) + 1;
    i3e = i3 + length(X_m) - 1;
    
    dv_u(i1:i1e) = gamma*(q_s(i1:i1e) - v_u(i1:i1e));
%     dv_l(i3:i3e) = -delta(i)*k_p*(v_l(i3:i3e)-rho*X_m) + delta(i)*k_i*w_l(i3:i3e);
    dv_l(i3:i3e) = -delta(i)*(v_l(i3:i3e)-rho*X_m);
%     dw_l(i3:i3e) = -delta(i)*k_i*(v_l(i3:i3e)-rho*X_m);
    dw_l(i3:i3e) = -w_l(i3:i3e);
    
    
    for j = 1 : SlaveRobotNum   %sigma, others
        i2 = (j-1) * SlaveRobotDOF + 1;
        i2e = i2 + SlaveRobotDOF - 1;
        i4 = (j-1) * length(X_m) + 1;
        i4e = i4 + length(X_m) -1;
    
        if adj(i, j) ~= 0
            %3.7
            dv_u(i1:i1e) = dv_u(i1:i1e) ...
                - adj(i,j)*(v_u(i1:i1e)-v_u(i2:i2e)) ...
                + adj(i,j)*(w_u(i1:i1e)-w_u(i2:i2e));
            %3.8
            dw_u(i1:i1e) = dw_u(i1:i1e) - adj(i,j)*(v_u(i1:i1e)-v_u(i2:i2e));
            %3.9
            dv_l(i3:i3e) = dv_l(i3:i3e) ...
                - adj(i,j)*(v_l(i3:i3e)-v_l(i4:i4e)) ...
                + adj(i,j)*(w_l(i3:i3e)-w_l(i4:i4e));
            %3.10
            dw_l(i3:i3e) = dw_l(i3:i3e) - adj(i,j)*(v_l(i3:i3e)-v_l(i4:i4e));
            
        end
    end
end

dv_u = dv_u * k_i;
dw_u = dw_u * k_i;
dv_l = dv_l * k_i;
dw_l = dw_l * k_i;

== matlab function distributed_system/swarm controller/MATLAB Function1 ==
  data: v_u input; u_f output; v_l input; q input; dq_s input
function u_f  = fcn(v_u, v_l, q, dq_s)
SlaveRobotNum = 6;
SlaveRobotDOF = 3;

q_d = zeros(length(q),1);
d_f = zeros(length(q),1);
d_f(1) = 1;
u_f = zeros(length(q),1);
k_f = 0.1;
k_fd = 0;

for i = 1 : SlaveRobotNum   %robot number
    %index
    i1 = (i-1) * SlaveRobotDOF + 1;
    i1e = i1 + SlaveRobotDOF - 1;
    i3 = (i-1) * (length(v_l)/SlaveRobotNum) + SlaveRobotDOF + 1;
    i3e = i3 + SlaveRobotDOF - 1;
    scaling = diag(v_l(i3:i3e));
    
    q_d(i1:i1e) = scaling*d_f(i1:i1e) + v_u(i1:i1e);
    u_f(i1:i1e) = -k_f*( q(i1:i1e)-q_d(i1:i1e) )- k_fd*dq_s(i1:i1e);
    
    if i ~= SlaveRobotNum
        d_f(i1+SlaveRobotDOF:i1e+SlaveRobotDOF) ...
            = rotz(360/SlaveRobotNum)*d_f(i1:i1e);
    end
end

== matlab function distributed_system/touch controller/control input ==
  data: Y_m_thetahat_m input; Jacobian input; s_m input; e_m input; u_m output; de_m input; dX_m input; u_m1 output; u_m2 output; u_m3 output; u_m4 output
function [u_m, u_m1,u_m2, u_m3, u_m4] = fcn(Y_m_thetahat_m, Jacobian, s_m, e_m, de_m, dX_m)
k_sm = diag([1;1.5;1.8]*40);
k_pm = diag([1.7;2.5;2.5]*10^(-4));
k_dm = diag([1.7;1.5;1.5]*10^(-3));
k_tm = diag([1;1;1]*10);
p_m = -k_tm*e_m + dX_m;
% u_m = Y_m_thetahat_m ...
%     - (k_sm + k_pm*Jacobian.'*Jacobian)*s_m ...
%     + k_dm*Jacobian.'*de_m;
u_m1 = Y_m_thetahat_m;
u_m2 = - k_sm*s_m;
u_m3 = - k_pm*Jacobian.'*p_m;
u_m4 = k_dm*Jacobian.'*de_m;
u_m = u_m1 + u_m2 + u_m3 + u_m4*0;

== matlab function distributed_system/touch controller/sliding ==
  data: invJacobian input; dinvJacobian input; e_m input; de_m input; dq_m input; s_m output; v_m output; a_m output
function [s_m, v_m, a_m] = fcn(invJacobian, dinvJacobian, e_m, de_m, dq_m)
k_tm = diag([1;1;1]*10);
s_m = -invJacobian*k_tm*e_m + dq_m;
v_m = dq_m - s_m;
a_m = dinvJacobian*k_tm*e_m + invJacobian*k_tm*de_m;

== matlab function distributed_system/touch controller/Y ==
  data: q input; Y output; dq input; v input; a input
function Y = fcn(q,dq,v,a)
%#codegen

Y11=a(1)*cos(2*q(2))-sin(2*q(2))*(v(2)*dq(1)-v(1)*dq(2));
Y12=-sin(2*q(2)+2*q(3))*dq(1)*(v(2)+v(3))-v(1)*sin(2*q(2)+2*q(3))*(dq(2)-dq(3))+a(1)*cos(2*q(2)+2*q(3));
Y13=a(1)*(sin(2*q(2)+ q(3))+sin(q(3)))+0.5*cos(q(3))*(v(1)*dq(3)+v(3)*dq(1))+cos(2*q(2)+q(3))*(v(2)*dq(1)+0.5*v(3)*dq(1)+v(1)*dq(2)+0.5*v(1)*dq(3));
Y14=a(1);
Y15=0;
Y16=0;
Y17=0;
Y18=0;

Y21=v(1)*sin(2*q(2))*dq(1);
Y22=v(1)*sin(2*q(2)+2*q(3))*dq(1);
Y23=sin(q(3))*(2*a(2)+a(3))-v(1)*cos(2*q(2)+q(3))*dq(1)+cos(q(3))*(v(3)*dq(2)+v(3)*dq(3)+v(2)*dq(3));
Y24=0;
Y25=a(2);
Y26=a(3);
Y27=sin(q(2)+q(3));
Y28=cos(q(2));


Y31=0;
Y32=v(1)*sin(2*q(2)+2*q(3))*dq(1);
Y33=a(2)*sin(q(3))-(0.5*v(1)*cos(2*q(2)+q(3))+0.5*v(1)*cos(q(3)))*dq(1)-cos(q(3))*v(2)*dq(2);
Y34=0;
Y35=0;
Y36=a(2)+a(3);
Y37=sin(q(2)+q(3));
Y38=0;

Y = [ Y11 Y21 Y31;
      Y12 Y22 Y32;
      Y13 Y23 Y33;
      Y14 Y24 Y34;
      Y15 Y25 Y35;
      Y16 Y26 Y36;
      Y17 Y27 Y37;
      Y18 Y28 Y38 ].';

== matlab function distributed_system/touch controller/dthetahat ==
  data: Y input; dthetahat output; s_m input
function dthetahat = fcn(Y, s_m)
%#codegen
dthetahat = -diag(ones(8,1)*0.1)*Y.'* s_m;

== matlab function distributed_system/touch controller/coordinate rotate1 ==
  data: u input; y output
function y = fcn(u)

y = roty(-90)*rotx(-90)*u;

== matlab function distributed_system/swarm controller/MATLAB Function2 ==
  data: dq_s input; u_es output; v_u input; v_l input
function u_es = fcn(dq_s, v_u, v_l)
SlaveRobotNum = 6;
SlaveRobotDOF = 3;
b = ones(SlaveRobotNum, 1)*0.3;
u_es = zeros(length(dq_s), 1);
Gamma = 0.1;
Lambda = 0.3;

for i = 1:SlaveRobotNum
%     index, 'e' for end
    i1 = (i-1) * SlaveRobotDOF + 1;
    i1e = i1 + SlaveRobotDOF - 1;
    i2 = (i-1) * (length(v_l)/SlaveRobotNum) + 1;
    i2e = i2 + SlaveRobotDOF - 1;   %leading G terms
    
    u_es(i1:i1e) = -b(i)*dq_s(i1:i1e) ...
        - eye(SlaveRobotDOF)*Gamma*(v_u(i1:i1e)-v_l(i2:i2e)) ...   %eye to be modified
        - Lambda * eye(SlaveRobotDOF) * dq_s(i1:i1e);
end

== matlab function distributed_system/swarm controller/MATLAB Function3 ==
  data: q input; u_a output
function u_a = fcn(q)

u_a = 0;

== matlab function distributed_system/swarm controller/adjecency ==
  data: adj output
% function adj = adjecency(q)
% SlaveRobotNum = 6;
% SlaveRobotDOF = 3;
% DistanceLimit = 10;
% 
% reachable = zeros(SlaveRobotNum, SlaveRobotNum);
% position = zeros(SlaveRobotNum, SlaveRobotDOF);
% 
% for num = 1 : SlaveRobotNum
%     for axis = 1 : SlaveRobotDOF
%         position(num, axis) = q( (num-1)*SlaveRobotDOF + axis);    
%     end
% end
% 
% for i = 1 : SlaveRobotNum
%     for j = 1 : SlaveRobotNum
%         
%         if i == j
%             reachable(i,j) = 0;
%         elseif norm(position(i,:) - position(j,:)) <= DistanceLimit
%             reachable(i,j) = 1;
%         else
%             reachable(i,j) = 0;
%         end
%     
%     end
% end
% 
% adj = reachable;

function adj = adjecency()
adj = [0 1 0 0 0 1;
       1 0 1 0 0 0;
       0 1 0 1 0 0;
       0 0 1 0 1 0;
       0 0 0 1 0 1;
       1 0 0 0 1 0;];

== matlab function distributed_system/swarm controller/coordinate rotate ==
  data: u input; y output
function y = fcn(u)
y = zeros(length(u),1);
% y(1:3) = rotx(90)*roty(90)*u(1:3);
% y(4:6) = rotx(90)*roty(90)*u(4:6);
y(1) = u(3);
y(2) = u(1);
y(3) = u(2);

y(4) = u(6);
y(5) = u(4);
y(6) = u(5);

== matlab function distributed_system/swarm controller/MATLAB Function4 ==
  data: X_s output; v_u input
function X_s = fcn(v_u)
% X_s = v_u(1:3);
X_s = v_u(4:6);

== matlab function distributed_system/touch controller/Jacobian ==
  data: q input; J output; dJ output; dq input; invJ output; dinvJ output
function [J, dJ, invJ, dinvJ] = fcn(q, dq)
%#codegen

L1=133;
L2=133;

q1 = q(1);
q2 = q(2);
q3 = q(3);

dq1 = dq(1);
dq2 = dq(2);
dq3 = dq(3);

j11 = -L1*cos( q1 )*cos( q2 ) - L2*cos( q1 )*cos( q2 )*sin( q3 ) - L2*cos( q1 )*sin( q2 )*cos( q3 );
j12 = L2*sin( q1 )*sin( q2 )*sin( q3 ) + L1*sin( q1 )*sin( q2 ) - L2*sin( q1 )*cos( q2 )*cos( q3 );
j13 = -L2*sin( q1 )*cos( q2 )*cos( q3 ) + L2*sin( q1 )*sin( q2 )*sin( q3 );
j22 = L2*sin( q2 )*cos( q3 ) + L2*cos( q2 )*sin( q3 ) + L1*cos( q2 );
j23 = L2*cos( q2 )*sin( q3 ) + L2*sin( q2 )*cos( q3 );
j31 = -L2*sin( q1 )*sin( q2 )*cos( q3 ) - L1*sin( q1 )*cos( q2 ) - L2*sin( q1 )*cos( q2 )*sin( q3 );
j32 = L2*cos( q1 )*cos( q2 )*cos( q3 ) - L2*cos( q1 )*sin( q2 )*sin( q3 ) - L1*cos( q1 )*sin( q2 );
j33 = L2*cos( q1 )*cos( q2 )*cos( q3 ) - L2*cos( q1 )*sin( q2 )*sin( q3 );

J = [ j11 j12 j13;
       0  j22 j23;
      j31 j32 j33];

dJ11=L1*dq1*cos( q2 )*sin( q1 ) + L1*dq2*cos( q1 )*sin( q2 ) - L2*dq2*cos( q1 )*cos( q2 )*cos( q3 ) - L2*dq3*cos( q1 )*cos( q2 )*cos( q3 ) + L2*dq1*cos( q2 )*sin( q1 )*sin( q3 ) + L2*dq1*cos( q3 )*sin( q1 )*sin( q2 ) + L2*dq2*cos( q1 )*sin( q2 )*sin( q3 ) + L2*dq3*cos( q1 )*sin( q2 )*sin( q3 );
dJ12=L1*dq1*cos( q1 )*sin( q2 ) + L1*dq2*cos( q2 )*sin( q1 ) - L2*dq1*cos( q1 )*cos( q2 )*cos( q3 ) + L2*dq1*cos( q1 )*sin( q2 )*sin( q3 ) + L2*dq2*cos( q2 )*sin( q1 )*sin( q3 ) + L2*dq2*cos( q3 )*sin( q1 )*sin( q2 ) + L2*dq3*cos( q2 )*sin( q1 )*sin( q3 ) + L2*dq3*cos( q3 )*sin( q1 )*sin( q2 );
dJ13=L2*dq1*cos( q1 )*sin( q2 )*sin( q3 ) - L2*dq1*cos( q1 )*cos( q2 )*cos( q3 ) + L2*dq2*cos( q2 )*sin( q1 )*sin( q3 ) + L2*dq2*cos( q3 )*sin( q1 )*sin( q2 ) + L2*dq3*cos( q2 )*sin( q1 )*sin( q3 ) + L2*dq3*cos( q3 )*sin( q1 )*sin( q2 );
dJ22=L2*dq2*cos( q2 )*cos( q3 ) - L1*dq2*sin( q2 ) + L2*dq3*cos( q2 )*cos( q3 ) - L2*dq2*sin( q2 )*sin( q3 ) - L2*dq3*sin( q2 )*sin( q3 );
dJ23=L2*dq2*cos( q2 )*cos( q3 ) + L2*dq3*cos( q2 )*cos( q3 ) - L2*dq2*sin( q2 )*sin( q3 ) - L2*dq3*sin( q2 )*sin( q3 );
dJ31=L1*dq2*sin( q1 )*sin( q2 ) - L1*dq1*cos( q1 )*cos( q2 ) - L2*dq1*cos( q1 )*cos( q2 )*sin( q3 ) - L2*dq1*cos( q1 )*cos( q3 )*sin( q2 ) - L2*dq2*cos( q2 )*cos( q3 )*sin( q1 ) - L2*dq3*cos( q2 )*cos( q3 )*sin( q1 ) + L2*dq2*sin( q1 )*sin( q2 )*sin( q3 ) + L2*dq3*sin( q1 )*sin( q2 )*sin( q3 );
dJ32=L1*dq1*sin( q1 )*sin( q2 ) - L1*dq2*cos( q1 )*cos( q2 ) - L2*dq1*cos( q2 )*cos( q3 )*sin( q1 ) - L2*dq2*cos( q1 )*cos( q2 )*sin( q3 ) - L2*dq2*cos( q1 )*cos( q3 )*sin( q2 ) - L2*dq3*cos( q1 )*cos( q2 )*sin( q3 ) - L2*dq3*cos( q1 )*cos( q3 )*sin( q2 ) + L2*dq1*sin( q1 )*sin( q2 )*sin( q3 );
dJ33=L2*dq1*sin( q1 )*sin( q2 )*sin( q3 ) - L2*dq2*cos( q1 )*cos( q2 )*sin( q3 ) - L2*dq2*cos( q1 )*cos( q3 )*sin( q2 ) - L2*dq3*cos( q1 )*cos( q2 )*sin( q3 ) - L2*dq3*cos( q1 )*cos( q3 )*sin( q2 ) - L2*dq1*cos( q2 )*cos( q3 )*sin( q1 );

dJ= [dJ11 dJ12 dJ13;
     0    dJ22 dJ23;
     dJ31 dJ32 dJ33];
 
invJ = pinv(J);

dinvJ11 = (sin(q1)*dq1)/(L1*cos(q1)^2*cos(q2) + L1*cos(q2)*sin(q1)^2 + L2*cos(q2)*sin(q1)^2*sin(q3) + L2*cos(q3)*sin(q1)^2*sin(q2) + L2*cos(q1)^2*cos(q2)*sin(q3) + L2*cos(q1)^2*cos(q3)*sin(q2)) - (cos(q1)*(L1*cos(q1)^2*sin(q2)*dq2 + L1*sin(q1)^2*sin(q2)*dq2 - L2*cos(q1)^2*cos(q2)*cos(q3)*dq2 - L2*cos(q1)^2*cos(q2)*cos(q3)*dq3 - L2*cos(q2)*cos(q3)*sin(q1)^2*dq2 - L2*cos(q2)*cos(q3)*sin(q1)^2*dq3 + L2*cos(q1)^2*sin(q2)*sin(q3)*dq2 + L2*cos(q1)^2*sin(q2)*sin(q3)*dq3 + L2*sin(q1)^2*sin(q2)*sin(q3)*dq2 + L2*sin(q1)^2*sin(q2)*sin(q3)*dq3))/(L1*cos(q1)^2*cos(q2) + L1*cos(q2)*sin(q1)^2 + L2*cos(q2)*sin(q1)^2*sin(q3) + L2*cos(q3)*sin(q1)^2*sin(q2) + L2*cos(q1)^2*cos(q2)*sin(q3) + L2*cos(q1)^2*cos(q3)*sin(q2))^2; 
dinvJ12 = 0;
dinvJ13 = - (cos(q1)*dq1)/(L1*cos(q1)^2*cos(q2) + L1*cos(q2)*sin(q1)^2 + L2*cos(q2)*sin(q1)^2*sin(q3) + L2*cos(q3)*sin(q1)^2*sin(q2) + L2*cos(q1)^2*cos(q2)*sin(q3) + L2*cos(q1)^2*cos(q3)*sin(q2)) - (sin(q1)*(L1*cos(q1)^2*sin(q2)*dq2 + L1*sin(q1)^2*sin(q2)*dq2 - L2*cos(q1)^2*cos(q2)*cos(q3)*dq2 - L2*cos(q1)^2*cos(q2)*cos(q3)*dq3 - L2*cos(q2)*cos(q3)*sin(q1)^2*dq2 - L2*cos(q2)*cos(q3)*sin(q1)^2*dq3 + L2*cos(q1)^2*sin(q2)*sin(q3)*dq2 + L2*cos(q1)^2*sin(q2)*sin(q3)*dq3 + L2*sin(q1)^2*sin(q2)*sin(q3)*dq2 + L2*sin(q1)^2*sin(q2)*sin(q3)*dq3))/(L1*cos(q1)^2*cos(q2) + L1*cos(q2)*sin(q1)^2 + L2*cos(q2)*sin(q1)^2*sin(q3) + L2*cos(q3)*sin(q1)^2*sin(q2) + L2*cos(q1)^2*cos(q2)*sin(q3) + L2*cos(q1)^2*cos(q3)*sin(q2))^2;
dinvJ21 = (sin(q1)*(cos(q2)*cos(q3)*dq2 + cos(q2)*cos(q3)*dq3 - sin(q2)*sin(q3)*dq2 - sin(q2)*sin(q3)*dq3))/(L1*cos(q3)*cos(q1)^2*cos(q2)^2 + L1*cos(q3)*cos(q1)^2*sin(q2)^2 + L1*cos(q3)*cos(q2)^2*sin(q1)^2 + L1*cos(q3)*sin(q1)^2*sin(q2)^2) + (sin(q1)*(cos(q2)*sin(q3) + cos(q3)*sin(q2))*(L1*sin(q3)*cos(q1)^2*cos(q2)^2*dq3 + L1*sin(q3)*cos(q1)^2*sin(q2)^2*dq3 + L1*sin(q3)*cos(q2)^2*sin(q1)^2*dq3 + L1*sin(q3)*sin(q1)^2*sin(q2)^2*dq3))/(L1*cos(q3)*cos(q1)^2*cos(q2)^2 + L1*cos(q3)*cos(q1)^2*sin(q2)^2 + L1*cos(q3)*cos(q2)^2*sin(q1)^2 + L1*cos(q3)*sin(q1)^2*sin(q2)^2)^2 + (cos(q1)*(cos(q2)*sin(q3) + cos(q3)*sin(q2))*dq1)/(L1*cos(q3)*cos(q1)^2*cos(q2)^2 + L1*cos(q3)*cos(q1)^2*sin(q2)^2 + L1*cos(q3)*cos(q2)^2*sin(q1)^2 + L1*cos(q3)*sin(q1)^2*sin(q2)^2);
dinvJ22 = - (cos(q2)*sin(q3)*dq2 + cos(q3)*sin(q2)*dq2 + cos(q2)*sin(q3)*dq3 + cos(q3)*sin(q2)*dq3)/(L1*cos(q3)*cos(q2)^2 + L1*cos(q3)*sin(q2)^2) - ((L1*sin(q3)*cos(q2)^2*dq3 + L1*sin(q3)*sin(q2)^2*dq3)*(sin(q2)*sin(q3) - cos(q2)*cos(q3)))/(L1*cos(q3)*cos(q2)^2 + L1*cos(q3)*sin(q2)^2)^2;
dinvJ23 = (sin(q1)*(cos(q2)*sin(q3) + cos(q3)*sin(q2))*dq1)/(L1*cos(q3)*cos(q1)^2*cos(q2)^2 + L1*cos(q3)*cos(q1)^2*sin(q2)^2 + L1*cos(q3)*cos(q2)^2*sin(q1)^2 + L1*cos(q3)*sin(q1)^2*sin(q2)^2) - (cos(q1)*(cos(q2)*cos(q3)*dq2 + cos(q2)*cos(q3)*dq3 - sin(q2)*sin(q3)*dq2 - sin(q2)*sin(q3)*dq3))/(L1*cos(q3)*cos(q1)^2*cos(q2)^2 + L1*cos(q3)*cos(q1)^2*sin(q2)^2 + L1*cos(q3)*cos(q2)^2*sin(q1)^2 + L1*cos(q3)*sin(q1)^2*sin(q2)^2) - (cos(q1)*(cos(q2)*sin(q3) + cos(q3)*sin(q2))*(L1*sin(q3)*cos(q1)^2*cos(q2)^2*dq3 + L1*sin(q3)*cos(q1)^2*sin(q2)^2*dq3 + L1*sin(q3)*cos(q2)^2*sin(q1)^2*dq3 + L1*sin(q3)*sin(q1)^2*sin(q2)^2*dq3))/(L1*cos(q3)*cos(q1)^2*cos(q2)^2 + L1*cos(q3)*cos(q1)^2*sin(q2)^2 + L1*cos(q3)*cos(q2)^2*sin(q1)^2 + L1*cos(q3)*sin(q1)^2*sin(q2)^2)^2;
dinvJ31 = - (L1*cos(q1)*cos(q2)*dq1 - L1*sin(q1)*sin(q2)*dq2 + L2*cos(q1)*cos(q2)*sin(q3)*dq1 + L2*cos(q1)*cos(q3)*sin(q2)*dq1 + L2*cos(q2)*cos(q3)*sin(q1)*dq2 + L2*cos(q2)*cos(q3)*sin(q1)*dq3 - L2*sin(q1)*sin(q2)*sin(q3)*dq2 - L2*sin(q1)*sin(q2)*sin(q3)*dq3)/(L1*L2*cos(q3)*cos(q1)^2*cos(q2)^2 + L1*L2*cos(q3)*cos(q1)^2*sin(q2)^2 + L1*L2*cos(q3)*cos(q2)^2*sin(q1)^2 + L1*L2*cos(q3)*sin(q1)^2*sin(q2)^2) - ((L1*cos(q2)*sin(q1) + L2*cos(q2)*sin(q1)*sin(q3) + L2*cos(q3)*sin(q1)*sin(q2))*(L1*L2*sin(q3)*cos(q1)^2*cos(q2)^2*dq3 + L1*L2*sin(q3)*cos(q1)^2*sin(q2)^2*dq3 + L1*L2*sin(q3)*cos(q2)^2*sin(q1)^2*dq3 + L1*L2*sin(q3)*sin(q1)^2*sin(q2)^2*dq3))/(L1*L2*cos(q3)*cos(q1)^2*cos(q2)^2 + L1*L2*cos(q3)*cos(q1)^2*sin(q2)^2 + L1*L2*cos(q3)*cos(q2)^2*sin(q1)^2 + L1*L2*cos(q3)*sin(q1)^2*sin(q2)^2)^2;
dinvJ32 = (L1*cos(q2)*dq2 + L2*cos(q2)*sin(q3)*dq2 + L2*cos(q3)*sin(q2)*dq2 + L2*cos(q2)*sin(q3)*dq3 + L2*cos(q3)*sin(q2)*dq3)/(L1*L2*cos(q3)*cos(q2)^2 + L1*L2*cos(q3)*sin(q2)^2) + ((L1*L2*sin(q3)*cos(q2)^2*dq3 + L1*L2*sin(q3)*sin(q2)^2*dq3)*(L1*sin(q2) - L2*cos(q2)*cos(q3) + L2*sin(q2)*sin(q3)))/(L1*L2*cos(q3)*cos(q2)^2 + L1*L2*cos(q3)*sin(q2)^2)^2;
dinvJ33 = ((L1*cos(q1)*cos(q2) + L2*cos(q1)*cos(q2)*sin(q3) + L2*cos(q1)*cos(q3)*sin(q2))*(L1*L2*sin(q3)*cos(q1)^2*cos(q2)^2*dq3 + L1*L2*sin(q3)*cos(q1)^2*sin(q2)^2*dq3 + L1*L2*sin(q3)*cos(q2)^2*sin(q1)^2*dq3 + L1*L2*sin(q3)*sin(q1)^2*sin(q2)^2*dq3))/(L1*L2*cos(q3)*cos(q1)^2*cos(q2)^2 + L1*L2*cos(q3)*cos(q1)^2*sin(q2)^2 + L1*L2*cos(q3)*cos(q2)^2*sin(q1)^2 + L1*L2*cos(q3)*sin(q1)^2*sin(q2)^2)^2 - (L1*cos(q2)*sin(q1)*dq1 + L1*cos(q1)*sin(q2)*dq2 - L2*cos(q1)*cos(q2)*cos(q3)*dq2 - L2*cos(q1)*cos(q2)*cos(q3)*dq3 + L2*cos(q2)*sin(q1)*sin(q3)*dq1 + L2*cos(q3)*sin(q1)*sin(q2)*dq1 + L2*cos(q1)*sin(q2)*sin(q3)*dq2 + L2*cos(q1)*sin(q2)*sin(q3)*dq3)/(L1*L2*cos(q3)*cos(q1)^2*cos(q2)^2 + L1*L2*cos(q3)*cos(q1)^2*sin(q2)^2 + L1*L2*cos(q3)*cos(q2)^2*sin(q1)^2 + L1*L2*cos(q3)*sin(q1)^2*sin(q2)^2);

dinvJ = ...
    [dinvJ11 dinvJ12 dinvJ13;
    dinvJ21 dinvJ22 dinvJ23;
    dinvJ31 dinvJ32 dinvJ33];
